simulink model "model"  (R2023b)
settings: Solver=VariableStepAuto  StartTime=0.0  StopTime=10.0  RelTol=1e-3
undefined symbols (not defined in the file): DiscIntNeverNeededParam, Newton, Raphson
libraries: simulink x46, slpidlib x9
(part 1 of 2)
settings Model: Creator=OSCAR4  LastModifiedBy=ojiken

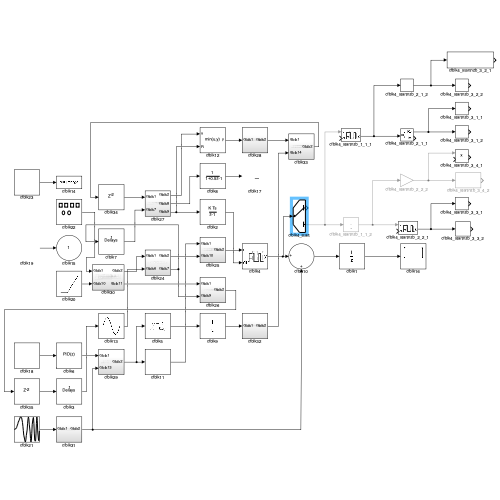
[thumbnail: Simulink's stored preview of the top-level diagram]
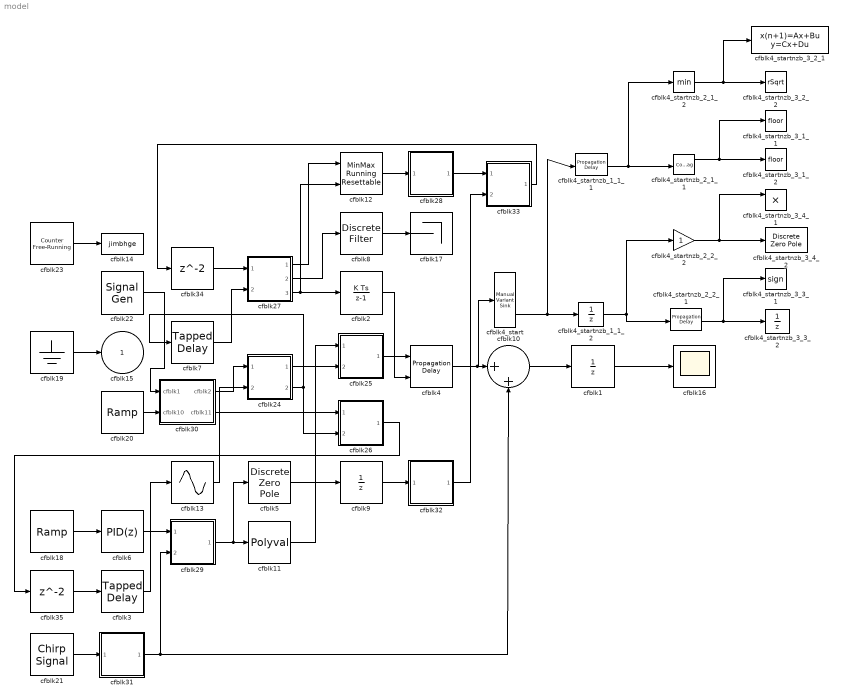
== system model ==
  cfblk1 : UnitDelay  HasFrameUpgradeWarning=on
  cfblk10 : Sum  Inputs=|++
  cfblk11 : Polyval  Coefs=[ +2.081618890e-019, -1.441693666e-014, +4.719686976e-010, -8.536869453e-006, +1.621573104e-001, -8.087801117e+001 ]
  cfblk12 : simulink/Math Operations/MinMax Running Resettable  Function=min  vinit=0.0
  cfblk13 : Sin  TimeSource=Use external signal  SampleTime=0
  cfblk14 : ToWorkspace  VariableName=jimbhge  SaveFormat=Timeseries  SampleTime=-1
  cfblk16 : Scope
  cfblk17 : Terminator
  cfblk18 : simulink/Sources/Ramp  slope=[-2549.980558]  start=[17.465354]  InitialOutput=[-530304.181969]
  cfblk19 : Ground
  cfblk2 : DiscreteIntegrator  ICPrevOutput=DiscIntNeverNeededParam  ICPrevScaledInput=DiscIntNeverNeededParam
  cfblk20 : simulink/Sources/Ramp  slope=[-906.393832]  start=[32.590534]  InitialOutput=[-89709.593460]
  cfblk21 : simulink/Sources/Chirp Signal  f1=[-269408375.768140]  T=[449577602.618100]  f2=[513643187.396250]
  cfblk22 : SignalGenerator  WaveForm=square  Amplitude=[544340339.779621]
  cfblk23 : simulink/Sources/Counter Free-Running  NumBits=[42.000000]  tsamp=-1
  cfblk24 : Subsystem
  cfblk25 : Subsystem
  cfblk26 : Subsystem
  cfblk27 : Subsystem
  cfblk28 : Subsystem
  cfblk29 : Subsystem
  cfblk3 : simulink/Discrete/Tapped Delay  vinit=0.0  samptime=-1  NumDelays=1  DelayOrder=Oldest  includeCurrent=off
  cfblk30 : Subsystem
  cfblk31 : Subsystem
  cfblk32 : Subsystem
  cfblk33 : Subsystem
  cfblk34 : Delay  SampleTime=1
  cfblk35 : Delay  SampleTime=1
  cfblk4 : PropagationDelay  SampleTime=1
  cfblk4_start : simulink/Signal Routing/Manual Variant Sink  NumChoices=2  LabelModeActiveChoice=V_1
  cfblk4_startnzb_1_1_1 : PropagationDelay
  cfblk4_startnzb_1_1_2 : UnitDelay  SampleTime=-1  HasFrameUpgradeWarning=on
  cfblk4_startnzb_2_1_1 : ComplexToRealImag
  cfblk4_startnzb_2_1_2 : MinMax
  cfblk4_startnzb_2_2_1 : PropagationDelay
  cfblk4_startnzb_2_2_2 : Gain
  cfblk4_startnzb_3_1_1 : Rounding
  cfblk4_startnzb_3_1_2 : Rounding
  cfblk4_startnzb_3_2_1 : DiscreteStateSpace  SampleTime=-1
  cfblk4_startnzb_3_2_2 : Sqrt  Operator=rSqrt
  cfblk4_startnzb_3_3_1 : Signum
  cfblk4_startnzb_3_3_2 : UnitDelay  SampleTime=-1  HasFrameUpgradeWarning=on
  cfblk4_startnzb_3_4_1 : Product
  cfblk4_startnzb_3_4_2 : DiscreteZeroPole  Poles=[0 0.5]  Gain=1  SampleTime=-1
  cfblk5 : DiscreteZeroPole  Poles=[0 0.5]  Gain=1
  cfblk6 : slpidlib/PID Controller  Controller=PID  Form=Parallel  TimeDomain=Discrete-time  UseExternalTs=off  SampleTime=1  IntegratorMethod=Forward Euler  FilterMethod=Forward Euler  ControllerParametersSource=internal  P=1  I=1  UseKiTs=off  D=0  N=100  UseFilter=on  TunerSelectOption=Transfer Function Based (PID Tuner App)  InitialConditionSource=internal  InitialConditionForIntegrator=0  InitialConditionForFilter=0  DifferentiatorICPrevScaledInput=0  ExternalReset=none  TrackingMode=off  Kt=1  LimitOutput=off  SatLimitsSource=internal  UpperSaturationLimit=inf  LowerSaturationLimit=-inf  LinearizeAsGain=off  AntiWindupMode=none  Kb=1  LimitIntegrator=off  UpperIntegratorSaturationLimit=inf  LowerIntegratorSaturationLimit=-inf  POutMin=[]  POutMax=[]  IOutMin=[]  IOutMax=[]  DOutMin=[]  DOutMax=[]  NOutMin=[]  NOutMax=[]  SumOutMin=[]  SumOutMax=[]  SaturationOutMin=[]  SaturationOutMax=[]  PParamMin=[]  PParamMax=[]  IParamMin=[]  IParamMax=[]  DParamMin=[]  DParamMax=[]  NParamMin=[]  NParamMax=[]  KbParamMin=[]  KbParamMax=[]  KtParamMin=[]  KtParamMax=[]  KbOutMin=[]  KbOutMax=[]  KtOutMin=[]  KtOutMax=[]  IntegratorOutMin=[]  IntegratorOutMax=[]  FilterOutMin=[]  FilterOutMax=[]  SumI1OutMin=[]  SumI1OutMax=[]  SumI2OutMin=[]  SumI2OutMax=[]  SumI3OutMin=[]  SumI3OutMax=[]  SumI4OutMin=[]  SumI4OutMax=[]  SumDOutMin=[]  SumDOutMax=[]  DifferentiatorOutMin=[]  DifferentiatorOutMax=[]  FilterDiffOutCoefMin=[]  FilterDiffOutCoefMax=[]  ReciprocalOutMin=[]  ReciprocalOutMax=[]  SumDenOutMin=[]  SumDenOutMax=[]  SumNumOutMin=[]  SumNumOutMax=[]  DivideOutMin=[]  DivideOutMax=[]  UdiffTsProdOutMin=[]  UdiffTsProdOutMax=[]  NTsProdOutMin=[]  NTsProdOutMax=[]  UintegralTsProdOutMin=[]  UintegralTsProdOutMax=[]  UngainTsProdOutMin=[]  UngainTsProdOutMax=[]  ClampingZeroOutDataTypeStr=Inherit: Inherit via back propagation  ClampingZeroOutMin=[]  ClampingZeroOutMax=[]  FilterDenConstantOutDataTypeStr=Inherit: Inherit via back propagation  FilterDenConstantOutMin=[]  FilterDenConstantOutMax=[]  PCopyOutDataTypeStr=Inherit: Inherit via back propagation  PCopyOutMin=[]  PCopyOutMax=[]  NCopyOutDataTypeStr=Inherit: Inherit via back propagation  NCopyOutMin=[]  NCopyOutMax=[]  IntegratorContinuousStateAttributes=''  IntegratorStateMustResolveToSignalObject=off  IntegratorRTWStateStorageClass=Auto  FilterContinuousStateAttributes=''  FilterStateMustResolveToSignalObject=off  FilterRTWStateStorageClass=Auto  ParallelPVariant=InternalParameters  IdealPVariant=Disabled  IVariant=InternalParameters  DVariant=InternalParameters  IntegratorVariant=Discrete  SatVariant=Disabled  AWVariant=Passthrough  PCopyVariant=Disabled  TRVariant=Disabled  FdbkBlocksVariant=Forward  IdealPFdbkVariant=Disabled  SatFdbkVariant=Disabled  DerivativeFilterVariant=ForwardEulerFilter  NVariant=InternalParameters  NCopyVariant=Disabled  FilterICVariant=InternalICsFilter  IntegratorICVariant=InternalICs  ExternalResetVariant=Disabled  TRSumVariant=Passthrough  SumFdbkVariant=Disabled  SumVariant=Sum_PID  TsampFilterVariant=InternalTs  TsampNgainVariant=Passthrough  TsampIntegralVariant=Disabled_SignalSpec  ExternalSaturationOutDataTypeStr=Inherit: Same as second input
      settings: LibrarySourceBlock=simulink/Discrete/Discrete PID Controller
  cfblk7 : simulink/Discrete/Tapped Delay  vinit=0.0  samptime=-1  NumDelays=1  DelayOrder=Oldest  includeCurrent=off
  cfblk8 : DiscreteFilter  SampleTime=1
  cfblk9 : UnitDelay  HasFrameUpgradeWarning=on
  cfblk15 : Outport
  wires:
  cfblk4_startnzb_2_2_2/1 -> cfblk4_startnzb_3_4_2/1, cfblk4_startnzb_3_4_1/1
  cfblk4_startnzb_2_1_2/1 -> cfblk4_startnzb_3_2_2/1, cfblk4_startnzb_3_2_1/1
  cfblk10/1 -> cfblk1/1
  cfblk33/1(cfblk2) -> cfblk34/1
  cfblk4_startnzb_1_1_2/1 -> cfblk4_startnzb_2_2_2/1, cfblk4_startnzb_2_2_1/1
  cfblk32/1(cfblk2) -> cfblk33/2(cfblk14)
  cfblk4/1 -> cfblk4_start/1, cfblk10/1
  cfblk28/1(cfblk2) -> cfblk33/1(cfblk1)
  cfblk9/1 -> cfblk32/1(cfblk1)
  cfblk2/1 -> cfblk4/2
  cfblk26/1(cfblk2) -> cfblk35/1
  cfblk8/1 -> cfblk17/1
  cfblk4_startnzb_1_1_1/1 -> cfblk4_startnzb_2_1_2/1, cfblk4_startnzb_2_1_1/1
  cfblk12/1 -> cfblk28/1(cfblk1)
  cfblk24/2(cfblk7) -> cfblk26/2(cfblk9), cfblk7/1
  cfblk30/2(cfblk11) -> cfblk26/1(cfblk1)
  cfblk27/2(cfblk8) -> cfblk8/1
  cfblk5/1 -> cfblk9/1
  cfblk27/3(cfblk9) -> cfblk2/1, cfblk12/2
  cfblk30/1(cfblk2) -> cfblk24/1(cfblk1)
  cfblk4_start/2 -> cfblk4_startnzb_1_1_2/1, cfblk4_startnzb_1_1_1/1
  cfblk7/1 -> cfblk27/2(cfblk7)
  cfblk4_startnzb_2_2_1/1 -> cfblk4_startnzb_3_3_2/1, cfblk4_startnzb_3_3_1/1
  cfblk24/1(cfblk2) -> cfblk25/2(cfblk10)
  cfblk34/1 -> cfblk27/1(cfblk1)
  cfblk20/1 -> cfblk30/2(cfblk10)
  cfblk13/1 -> cfblk24/2(cfblk6)
  cfblk18/1 -> cfblk6/1
  cfblk6/1 -> cfblk29/1(cfblk1)
  cfblk31/1(cfblk2) -> cfblk29/2(cfblk13), cfblk10/2
  cfblk23/1 -> cfblk14/1
  cfblk22/1 -> cfblk30/1(cfblk1)
  cfblk3/1 -> cfblk13/1
  cfblk27/1(cfblk2) -> cfblk12/1
  cfblk4_startnzb_2_1_1/1 -> cfblk4_startnzb_3_1_2/1, cfblk4_startnzb_3_1_1/1
  cfblk21/1 -> cfblk31/1(cfblk1)
  cfblk25/1(cfblk2) -> cfblk4/1
  cfblk35/1 -> cfblk3/1
  cfblk29/1(cfblk2) -> cfblk5/1, cfblk11/1
  cfblk19/1 -> cfblk15/1
  cfblk1/1 -> cfblk16/1
  cfblk11/1 -> cfblk25/1(cfblk1)

== system model/cfblk24 ==
  cfblk1 : Inport
  cfblk6 : Inport  Port=2
  cfblk3 : DiscreteFir  SampleTime=1
  cfblk4 : Constant  Value=[619260692.211267]  SampleTime=1
  cfblk5 : Constant  Value=[619560780.626358]  SampleTime=1
  cfblk2 : Outport
  cfblk7 : Outport  Port=2
  wires:
  cfblk6/1 -> cfblk3/1
  cfblk3/1 -> cfblk7/1
  cfblk4/1 -> cfblk2/1

== system model/cfblk25 ==
  cfblk1 : Inport
  cfblk10 : Inport  Port=2
  cfblk{11..14} (4 alike) : Delay  SampleTime=1
  cfblk3 : simulink/Discrete/Transfer Fcn Real Zero  ZeroZ=0.75  ICPrevInput=0.0  DoSatur=off
  cfblk4 : UnaryMinus
  cfblk5 : Subsystem
  cfblk6 : Subsystem
  cfblk7 : Subsystem
  cfblk8 : Subsystem
  cfblk9 : Subsystem
  cfblk2 : Outport
  wires:
  cfblk10/1 -> cfblk5/1(cfblk1)
  cfblk6/1(cfblk2) -> cfblk2/1, cfblk13/1
  cfblk8/2(cfblk11) -> cfblk3/1
  cfblk1/1 -> cfblk7/1(cfblk1), cfblk5/5(cfblk15)
  cfblk7/1(cfblk2) -> cfblk5/4(cfblk14), cfblk8/3(cfblk10)
  cfblk5/1(cfblk2) -> cfblk4/1
  cfblk4/1 -> cfblk8/1(cfblk1)
  cfblk9/1(cfblk2) -> cfblk6/1(cfblk1)
  cfblk3/1 -> cfblk9/1(cfblk1), cfblk12/1
  cfblk8/1(cfblk2) -> cfblk11/1
  cfblk11/1 -> cfblk5/3(cfblk13)
  cfblk12/1 -> cfblk8/2(cfblk9)
  cfblk13/1 -> cfblk5/2(cfblk12)
  cfblk5/2(cfblk16) -> cfblk14/1
  cfblk14/1 -> cfblk7/2(cfblk13)

== system model/cfblk26 ==
  cfblk1 : Inport
  cfblk9 : Inport  Port=2
  cfblk10 : Delay  SampleTime=1
  cfblk3 : DiscreteFilter  SampleTime=1
  cfblk4 : DiscreteIntegrator  ICPrevOutput=DiscIntNeverNeededParam  ICPrevScaledInput=DiscIntNeverNeededParam
  cfblk5 : simulink/Discrete/Transfer Fcn Real Zero  ZeroZ=0.75  ICPrevInput=0.0  DoSatur=off
  cfblk6 : Sum  Inputs=+-
  cfblk7 : Constant  Value=[-48546722.892624]  SampleTime=1
  cfblk8 : Subsystem
  cfblk2 : Outport
  wires:
  cfblk7/1 -> cfblk3/1
  cfblk3/1 -> cfblk8/1(cfblk1)
  cfblk9/1 -> cfblk4/1, cfblk8/4(cfblk13)
  cfblk4/1 -> cfblk6/1
  cfblk1/1 -> cfblk8/2(cfblk11)
  cfblk5/1 -> cfblk6/2
  cfblk8/1(cfblk2) -> cfblk5/1
  cfblk8/2(cfblk14) -> cfblk2/1
  cfblk6/1 -> cfblk10/1
  cfblk10/1 -> cfblk8/3(cfblk12)

== system model/cfblk27 ==
  cfblk1 : Inport
  cfblk7 : Inport  Port=2
  cfblk10 : Delay  SampleTime=1
  cfblk11 : Delay  SampleTime=1
  cfblk3 : Product  Inputs=*
  cfblk4 : Constant  Value=[-592211525.681612]  SampleTime=1
  cfblk5 : Subsystem
  cfblk6 : Subsystem
  cfblk2 : Outport
  cfblk8 : Outport  Port=2
  cfblk9 : Outport  Port=3
  wires:
  cfblk6/1(cfblk2) -> cfblk9/1
  cfblk7/1 -> cfblk2/1, cfblk8/1, cfblk6/3(cfblk12)
  cfblk5/1(cfblk2) -> cfblk3/1
  cfblk4/1 -> cfblk5/1(cfblk1), cfblk5/4(cfblk15), cfblk6/4(cfblk13)
  cfblk3/1 -> cfblk10/1, cfblk11/1
  cfblk1/1 -> cfblk6/2(cfblk11), cfblk5/6(cfblk17)
  cfblk6/2(cfblk15) -> cfblk5/2(cfblk13)
  cfblk6/3(cfblk16) -> cfblk5/3(cfblk14), cfblk5/5(cfblk16)
  cfblk10/1 -> cfblk6/1(cfblk1)
  cfblk11/1 -> cfblk6/5(cfblk14)

== system model/cfblk28 ==
  cfblk1 : Inport
  cfblk10 : Subsystem
  cfblk11 : Subsystem
  cfblk{12..15} (4 alike) : Delay  SampleTime=1
  cfblk3 : Delay  DelayLengthSource=Input port  SampleTime=1
      settings: InputPortMap=u0,p1
  cfblk4 : UnitDelay  HasFrameUpgradeWarning=on
  cfblk5 : Rounding
  cfblk6 : MinMax  Inputs=3
  cfblk7 : DotProduct  OutDataTypeStr=Inherit: Inherit via internal rule
  cfblk8 : Product  Inputs=**
  cfblk9 : Constant  Value=[-543142463.220039]  SampleTime=1
  cfblk2 : Outport
  wires:
  cfblk1/1 -> cfblk6/1
  cfblk9/1 -> cfblk10/1(cfblk1), cfblk11/1(cfblk1), cfblk11/3(cfblk13)
  cfblk3/1 -> cfblk10/2(cfblk14), cfblk2/1
  cfblk5/1 -> cfblk10/4(cfblk16), cfblk14/1
  cfblk6/1 -> cfblk8/2, cfblk3/1
  cfblk11/1(cfblk2) -> cfblk5/1, cfblk3/2, cfblk13/1
  cfblk8/1 -> cfblk4/1, cfblk11/2(cfblk12)
  cfblk10/1(cfblk2) -> cfblk7/1
  cfblk10/2(cfblk17) -> cfblk7/2
  cfblk4/1 -> cfblk12/1
  cfblk12/1 -> cfblk6/2
  cfblk13/1 -> cfblk6/3
  cfblk14/1 -> cfblk8/1
  cfblk7/1 -> cfblk15/1
  cfblk15/1 -> cfblk10/3(cfblk15)

== system model/cfblk29 ==
  cfblk1 : Inport
  cfblk13 : Inport  Port=2
  cfblk10 : Constant  Value=[-634116043.235819]  SampleTime=1
  cfblk11 : Subsystem
  cfblk12 : Subsystem
  cfblk14 : Delay  SampleTime=1
  cfblk3 : DiscreteFir  SampleTime=1
  cfblk4 : DiscreteStateSpace
  cfblk5 : simulink/Discrete/Transfer Fcn Lead or Lag  PoleZ=0.95  ZeroZ=0.75  ICPrevOutput=0.0  ICPrevInput=0.0  DoSatur=off
  cfblk6 : simulink/Math Operations/Slider Gain  gain=1  low=0  high=2
  cfblk7 : ComplexToRealImag
  cfblk8 : Squeeze
  cfblk9 : ComplexToMagnitudeAngle
  cfblk2 : Outport
  wires:
  cfblk4/1 -> cfblk2/1
  cfblk11/1(cfblk2) -> cfblk8/1
  cfblk7/1 -> cfblk12/1(cfblk1)
  cfblk10/1 -> cfblk5/1
  cfblk7/2 -> cfblk11/1(cfblk1)
  cfblk8/1 -> cfblk9/1
  cfblk3/1 -> cfblk7/1
  cfblk5/1 -> cfblk6/1
  cfblk9/1 -> cfblk4/1
  cfblk6/1 -> cfblk3/1
  cfblk12/1(cfblk2) -> cfblk11/3(cfblk8)
  cfblk9/2 -> cfblk14/1
  cfblk14/1 -> cfblk11/2(cfblk7)

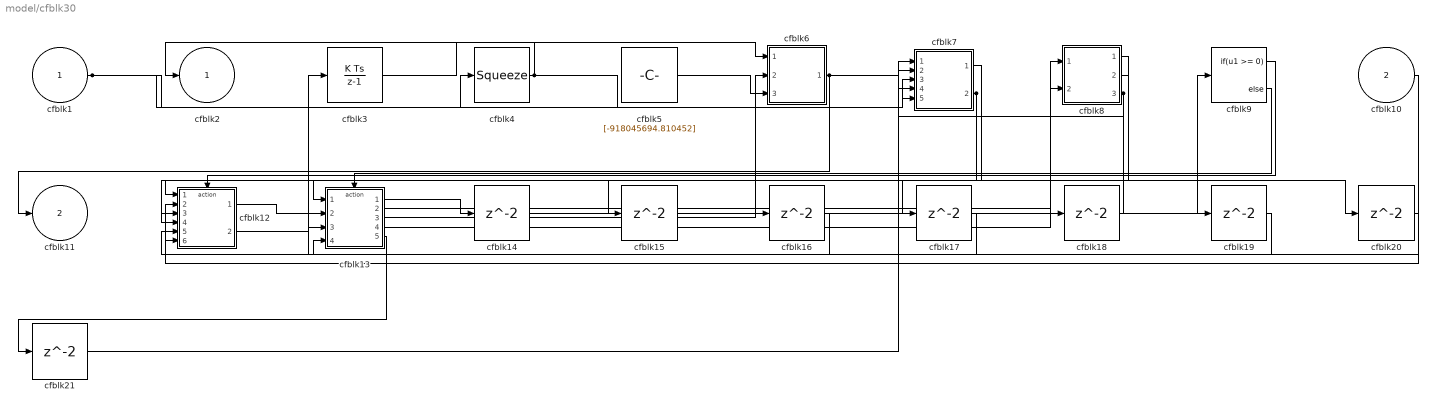
== system model/cfblk30 ==
  cfblk1 : Inport
  cfblk10 : Inport  Port=2
  cfblk12 : Subsystem  TreatAsAtomicUnit=on
  cfblk13 : Subsystem  TreatAsAtomicUnit=on
  cfblk{14..21} (8 alike) : Delay  SampleTime=1
  cfblk3 : DiscreteIntegrator  ICPrevOutput=DiscIntNeverNeededParam  ICPrevScaledInput=DiscIntNeverNeededParam
  cfblk4 : Squeeze
  cfblk5 : Constant  Value=[-918045694.810452]  SampleTime=1
  cfblk6 : Subsystem
  cfblk7 : Subsystem
  cfblk8 : Subsystem
  cfblk9 : If  IfExpression=u1 >= 0  SampleTime=1
  cfblk2 : Outport
  cfblk11 : Outport  Port=2
  wires:
  cfblk7/1(cfblk2) -> cfblk12/1(cfblk1)
  cfblk6/1(cfblk2) -> cfblk11/1, cfblk19/1, cfblk20/1
  cfblk4/1 -> cfblk2/1, cfblk7/3(cfblk13)
  cfblk7/2(cfblk16) -> cfblk13/1(cfblk1), cfblk12/3(cfblk11), cfblk12/4(cfblk12)
  cfblk1/1 -> cfblk4/1, cfblk7/5(cfblk15)
  cfblk3/1 -> cfblk6/1(cfblk1)
  cfblk13/2(cfblk14) -> cfblk8/1(cfblk1)
  cfblk13/3(cfblk15) -> cfblk6/2(cfblk10)
  cfblk5/1 -> cfblk6/3(cfblk11)
  cfblk12/1(cfblk2) -> cfblk13/2(cfblk11)
  cfblk12/2(cfblk15) -> cfblk3/1
  cfblk13/4(cfblk16) -> cfblk8/2(cfblk13)
  cfblk8/3(cfblk15) -> cfblk17/1, cfblk18/1
  cfblk10/1 -> cfblk12/2(cfblk10)
  cfblk9/1 -> cfblk12/Action
  cfblk9/2 -> cfblk13/Action
  cfblk13/1(cfblk2) -> cfblk14/1
  cfblk14/1 -> cfblk7/1(cfblk1)
  cfblk8/1(cfblk2) -> cfblk15/1
  cfblk15/1 -> cfblk9/1
  cfblk8/2(cfblk14) -> cfblk16/1
  cfblk16/1 -> cfblk13/3(cfblk12)
  cfblk17/1 -> cfblk13/4(cfblk13)
  cfblk18/1 -> cfblk7/4(cfblk14)
  cfblk19/1 -> cfblk12/5(cfblk13)
  cfblk20/1 -> cfblk12/6(cfblk14)
  cfblk13/5(cfblk17) -> cfblk21/1
  cfblk21/1 -> cfblk7/2(cfblk12)

== system model/cfblk31 ==
  cfblk1 : Inport
  cfblk3 : DiscreteFilter  SampleTime=1
  cfblk4 : simulink/Discrete/Tapped Delay  vinit=0.0  samptime=-1  NumDelays=1  DelayOrder=Oldest  includeCurrent=off
  cfblk5 : simulink/Discrete/Difference  ICPrevInput=0.0  OutMin=[]  OutMax=[]  OutDataTypeStr=Inherit: Inherit via back propagation  OutDataType=fixdt(1, 16)  OutScaling=2^-10  DoSatur=off
  cfblk6 : DiscreteFir  SampleTime=1
  cfblk7 : Math  Operator=pow
  cfblk8 : Product  Inputs=*
  cfblk2 : Outport
  wires:
  cfblk4/1 -> cfblk7/1
  cfblk1/1 -> cfblk6/1
  cfblk5/1 -> cfblk4/1
  cfblk6/1 -> cfblk5/1, cfblk3/1
  cfblk7/1 -> cfblk8/1
  cfblk8/1 -> cfblk2/1
  cfblk3/1 -> cfblk7/2

== system model/cfblk32 ==
  cfblk1 : Inport
  cfblk10 : Subsystem
  cfblk11 : Subsystem
  cfblk12 : Delay  SampleTime=1
  cfblk13 : Delay  SampleTime=1
  cfblk14 : Delay  SampleTime=1
  cfblk3 : simulink/Discrete/Transfer Fcn Lead or Lag  PoleZ=0.95  ZeroZ=0.75  ICPrevOutput=0.0  ICPrevInput=0.0  DoSatur=off
  cfblk4 : DotProduct  OutDataTypeStr=Inherit: Inherit via internal rule
  cfblk5 : Gain  Gain=[-290399110.976152]
  cfblk6 : Sin  TimeSource=Use external signal  SampleTime=0
  cfblk7 : Constant  Value=[164625169.803673]  SampleTime=1
  cfblk8 : Constant  Value=[629483974.627171]  SampleTime=1
  cfblk9 : Subsystem
  cfblk2 : Outport
  wires:
  cfblk9/1(cfblk2) -> cfblk6/1
  cfblk10/1(cfblk2) -> cfblk11/1(cfblk1)
  cfblk3/1 -> cfblk13/1, cfblk14/1
  cfblk10/2(cfblk17) -> cfblk11/3(cfblk7)
  cfblk11/1(cfblk2) -> cfblk3/1
  cfblk7/1 -> cfblk4/1, cfblk9/4(cfblk11), cfblk10/3(cfblk12), cfblk10/6(cfblk15)
  cfblk4/1 -> cfblk5/1, cfblk10/4(cfblk13)
  cfblk9/2(cfblk12) -> cfblk10/1(cfblk1)
  cfblk5/1 -> cfblk2/1
  cfblk8/1 -> cfblk9/2(cfblk9)
  cfblk1/1 -> cfblk9/3(cfblk10), cfblk10/7(cfblk16)
  cfblk9/3(cfblk13) -> cfblk4/2
  cfblk9/4(cfblk14) -> cfblk10/2(cfblk11)
  cfblk6/1 -> cfblk12/1
  cfblk12/1 -> cfblk9/1(cfblk1)
  cfblk13/1 -> cfblk11/2(cfblk6)
  cfblk14/1 -> cfblk10/5(cfblk14)

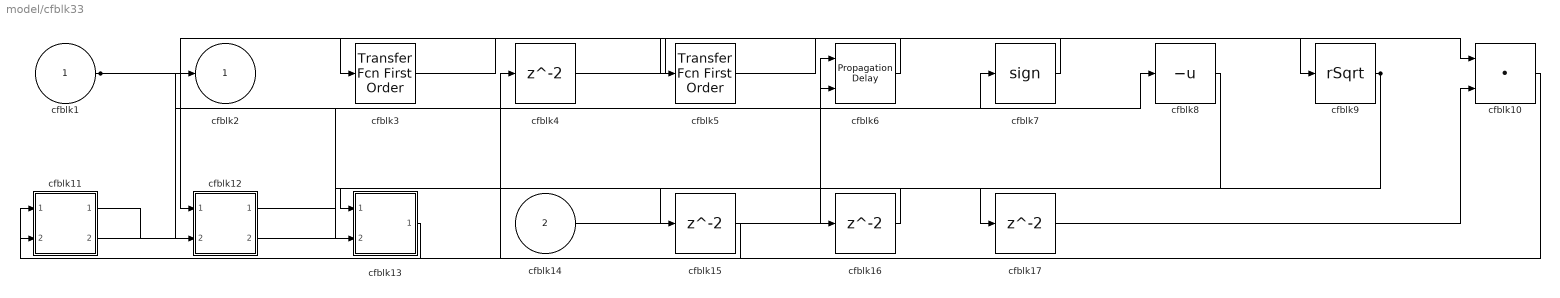
== system model/cfblk33 ==
  cfblk1 : Inport
  cfblk14 : Inport  Port=2
  cfblk10 : DotProduct  OutDataTypeStr=Inherit: Inherit via internal rule
  cfblk11 : Subsystem
  cfblk12 : Subsystem
  cfblk13 : Subsystem
  cfblk{4,15..17} (4 alike) : Delay  SampleTime=1
  cfblk3 : simulink/Discrete/Transfer Fcn First Order  PoleZ=0.95  ICPrevOutput=0.0  DoSatur=off
  cfblk5 : simulink/Discrete/Transfer Fcn First Order  PoleZ=0.95  ICPrevOutput=0.0  DoSatur=off
  cfblk6 : PropagationDelay  SampleTime=1
  cfblk7 : Signum
  cfblk8 : UnaryMinus
  cfblk9 : Sqrt  Operator=rSqrt  AlgorithmType=Newton-Raphson
  cfblk2 : Outport
  wires:
  cfblk14/1 -> cfblk6/1
  cfblk7/1 -> cfblk12/1(cfblk1)
  cfblk10/1 -> cfblk4/1
  cfblk6/1 -> cfblk3/1
  cfblk5/1 -> cfblk10/1
  cfblk4/1 -> cfblk9/1
  cfblk11/1(cfblk2) -> cfblk12/2(cfblk13)
  cfblk1/1 -> cfblk2/1, cfblk6/2
  cfblk11/2(cfblk7) -> cfblk7/1
  cfblk13/1(cfblk2) -> cfblk11/1(cfblk1)
  cfblk3/1 -> cfblk5/1
  cfblk12/2(cfblk14) -> cfblk8/1
  cfblk9/1 -> cfblk13/2(cfblk7), cfblk17/1
  cfblk12/1(cfblk2) -> cfblk15/1
  cfblk15/1 -> cfblk11/2(cfblk6)
  cfblk8/1 -> cfblk16/1
  cfblk16/1 -> cfblk13/1(cfblk1)
  cfblk17/1 -> cfblk10/2

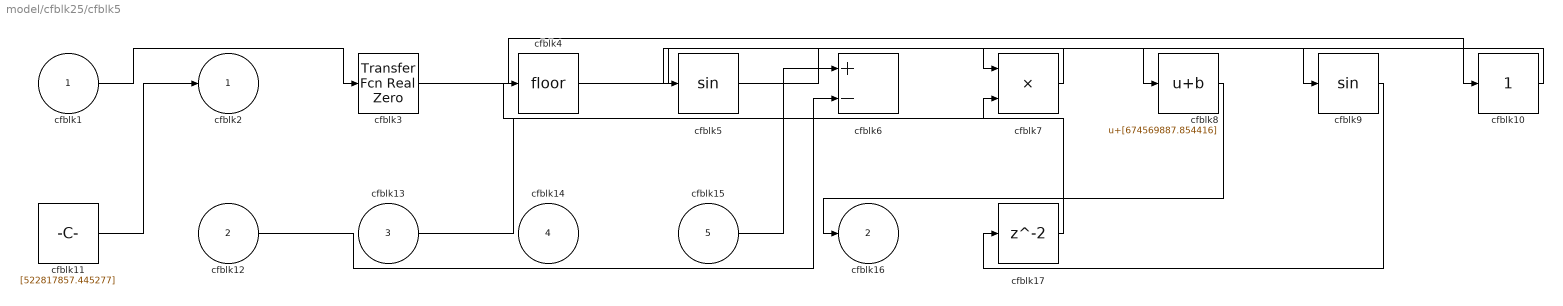
== system model/cfblk25/cfblk5 ==
  cfblk1 : Inport
  cfblk12 : Inport  Port=2
  cfblk13 : Inport  Port=3
  cfblk14 : Inport  Port=4
  cfblk15 : Inport  Port=5
  cfblk10 : simulink/Math Operations/Slider Gain  gain=1  low=0  high=2
  cfblk11 : Constant  Value=[522817857.445277]  SampleTime=1
  cfblk17 : Delay  SampleTime=1
  cfblk3 : simulink/Discrete/Transfer Fcn Real Zero  ZeroZ=0.75  ICPrevInput=0.0  DoSatur=off
  cfblk4 : Rounding
  cfblk5 : Trigonometry
  cfblk6 : Sum  Inputs=+-
  cfblk7 : Product
  cfblk8 : Bias  Bias=[674569887.854416]  SaturateOnIntegerOverflow=off
  cfblk9 : Trigonometry
  cfblk2 : Outport
  cfblk16 : Outport  Port=2
  wires:
  cfblk4/1 -> cfblk9/1
  cfblk11/1 -> cfblk2/1
  cfblk1/1 -> cfblk3/1
  cfblk15/1 -> cfblk6/1
  cfblk3/1 -> cfblk10/1
  cfblk7/1 -> cfblk5/1
  cfblk8/1 -> cfblk16/1
  cfblk12/1 -> cfblk6/2
  cfblk10/1 -> cfblk7/1
  cfblk13/1 -> cfblk7/2
  cfblk5/1 -> cfblk8/1
  cfblk9/1 -> cfblk17/1
  cfblk17/1 -> cfblk4/1

== system model/cfblk25/cfblk6 ==
  cfblk1 : Inport
  cfblk3 : DiscreteFir  SampleTime=1
  cfblk4 : simulink/Discrete/Difference  ICPrevInput=0.0  OutMin=[]  OutMax=[]  OutDataTypeStr=Inherit: Inherit via back propagation  OutDataType=fixdt(1, 16)  OutScaling=2^-10  DoSatur=off
  cfblk5 : Sum  Inputs=+-
  cfblk6 : Signum
  cfblk7 : Product
  cfblk8 : Rounding
  cfblk9 : Delay  SampleTime=1
  cfblk2 : Outport
  wires:
  cfblk3/1 -> cfblk8/1, cfblk7/2
  cfblk5/1 -> cfblk6/1
  cfblk1/1 -> cfblk5/2
  cfblk6/1 -> cfblk4/1, cfblk2/1
  cfblk4/1 -> cfblk3/1
  cfblk8/1 -> cfblk7/1
  cfblk7/1 -> cfblk9/1
  cfblk9/1 -> cfblk5/1

== system model/cfblk25/cfblk7 ==
  cfblk1 : Inport
  cfblk13 : Inport  Port=2
  cfblk10 : Abs  SaturateOnIntegerOverflow=off
  cfblk11 : Product
  cfblk12 : Constant  Value=[399015118.877011]  SampleTime=1
  cfblk14 : Delay  SampleTime=1
  cfblk15 : Delay  SampleTime=1
  cfblk3 : slpidlib/PID Controller  Controller=PID  Form=Parallel  TimeDomain=Discrete-time  UseExternalTs=off  SampleTime=1  IntegratorMethod=Forward Euler  FilterMethod=Forward Euler  ControllerParametersSource=internal  P=1  I=1  UseKiTs=off  D=0  N=100  UseFilter=on  TunerSelectOption=Transfer Function Based (PID Tuner App)  InitialConditionSource=internal  InitialConditionForIntegrator=0  InitialConditionForFilter=0  DifferentiatorICPrevScaledInput=0  ExternalReset=none  TrackingMode=off  Kt=1  LimitOutput=off  SatLimitsSource=internal  UpperSaturationLimit=inf  LowerSaturationLimit=-inf  LinearizeAsGain=off  AntiWindupMode=none  Kb=1  LimitIntegrator=off  UpperIntegratorSaturationLimit=inf  LowerIntegratorSaturationLimit=-inf  POutMin=[]  POutMax=[]  IOutMin=[]  IOutMax=[]  DOutMin=[]  DOutMax=[]  NOutMin=[]  NOutMax=[]  SumOutMin=[]  SumOutMax=[]  SaturationOutMin=[]  SaturationOutMax=[]  PParamMin=[]  PParamMax=[]  IParamMin=[]  IParamMax=[]  DParamMin=[]  DParamMax=[]  NParamMin=[]  NParamMax=[]  KbParamMin=[]  KbParamMax=[]  KtParamMin=[]  KtParamMax=[]  KbOutMin=[]  KbOutMax=[]  KtOutMin=[]  KtOutMax=[]  IntegratorOutMin=[]  IntegratorOutMax=[]  FilterOutMin=[]  FilterOutMax=[]  SumI1OutMin=[]  SumI1OutMax=[]  SumI2OutMin=[]  SumI2OutMax=[]  SumI3OutMin=[]  SumI3OutMax=[]  SumI4OutMin=[]  SumI4OutMax=[]  SumDOutMin=[]  SumDOutMax=[]  DifferentiatorOutMin=[]  DifferentiatorOutMax=[]  FilterDiffOutCoefMin=[]  FilterDiffOutCoefMax=[]  ReciprocalOutMin=[]  ReciprocalOutMax=[]  SumDenOutMin=[]  SumDenOutMax=[]  SumNumOutMin=[]  SumNumOutMax=[]  DivideOutMin=[]  DivideOutMax=[]  UdiffTsProdOutMin=[]  UdiffTsProdOutMax=[]  NTsProdOutMin=[]  NTsProdOutMax=[]  UintegralTsProdOutMin=[]  UintegralTsProdOutMax=[]  UngainTsProdOutMin=[]  UngainTsProdOutMax=[]  ClampingZeroOutDataTypeStr=Inherit: Inherit via back propagation  ClampingZeroOutMin=[]  ClampingZeroOutMax=[]  FilterDenConstantOutDataTypeStr=Inherit: Inherit via back propagation  FilterDenConstantOutMin=[]  FilterDenConstantOutMax=[]  PCopyOutDataTypeStr=Inherit: Inherit via back propagation  PCopyOutMin=[]  PCopyOutMax=[]  NCopyOutDataTypeStr=Inherit: Inherit via back propagation  NCopyOutMin=[]  NCopyOutMax=[]  IntegratorContinuousStateAttributes=''  IntegratorStateMustResolveToSignalObject=off  IntegratorRTWStateStorageClass=Auto  FilterContinuousStateAttributes=''  FilterStateMustResolveToSignalObject=off  FilterRTWStateStorageClass=Auto  ParallelPVariant=InternalParameters  IdealPVariant=Disabled  IVariant=InternalParameters  DVariant=InternalParameters  IntegratorVariant=Discrete  SatVariant=Disabled  AWVariant=Passthrough  PCopyVariant=Disabled  TRVariant=Disabled  FdbkBlocksVariant=Forward  IdealPFdbkVariant=Disabled  SatFdbkVariant=Disabled  DerivativeFilterVariant=ForwardEulerFilter  NVariant=InternalParameters  NCopyVariant=Disabled  FilterICVariant=InternalICsFilter  IntegratorICVariant=InternalICs  ExternalResetVariant=Disabled  TRSumVariant=Passthrough  SumFdbkVariant=Disabled  SumVariant=Sum_PID  TsampFilterVariant=InternalTs  TsampNgainVariant=Passthrough  TsampIntegralVariant=Disabled_SignalSpec  ExternalSaturationOutDataTypeStr=Inherit: Same as second input
      settings: LibrarySourceBlock=simulink/Discrete/Discrete PID Controller
  cfblk4 : simulink/Discrete/Transfer Fcn Lead or Lag  PoleZ=0.95  ZeroZ=0.75  ICPrevOutput=0.0  ICPrevInput=0.0  DoSatur=off
  cfblk5 : simulink/Discrete/Tapped Delay  vinit=0.0  samptime=-1  NumDelays=1  DelayOrder=Oldest  includeCurrent=off
  cfblk6 : Product
  cfblk7 : Product  Inputs=**
  cfblk8 : Sqrt  Operator=rSqrt  AlgorithmType=Newton-Raphson
  cfblk9 : Product  Inputs=**
  cfblk2 : Outport
  wires:
  cfblk3/1 -> cfblk10/1
  cfblk9/1 -> cfblk11/1
  cfblk10/1 -> cfblk7/1
  cfblk12/1 -> cfblk3/1
  cfblk1/1 -> cfblk6/1
  cfblk11/1 -> cfblk4/1
  cfblk4/1 -> cfblk7/2, cfblk15/1
  cfblk6/1 -> cfblk9/1
  cfblk5/1 -> cfblk8/1
  cfblk7/1 -> cfblk2/1, cfblk14/1
  cfblk8/1 -> cfblk9/2
  cfblk13/1 -> cfblk5/1
  cfblk14/1 -> cfblk6/2
  cfblk15/1 -> cfblk11/2

== system model/cfblk25/cfblk8 ==
  cfblk1 : Inport
  cfblk9 : Inport  Port=2
  cfblk10 : Inport  Port=3
  cfblk3 : simulink/Discrete/Tapped Delay  vinit=0.0  samptime=-1  NumDelays=1  DelayOrder=Oldest  includeCurrent=off
  cfblk4 : simulink/Discrete/Transfer Fcn Lead or Lag  PoleZ=0.95  ZeroZ=0.75  ICPrevOutput=0.0  ICPrevInput=0.0  DoSatur=off
  cfblk5 : PermuteDimensions
  cfblk6 : Signum
  cfblk7 : Constant  Value=[497245692.108561]  SampleTime=1
  cfblk8 : Constant  Value=[-352505690.659076]  SampleTime=1
  cfblk2 : Outport
  cfblk11 : Outport  Port=2
  wires:
  cfblk3/1 -> cfblk2/1
  cfblk9/1 -> cfblk4/1
  cfblk1/1 -> cfblk5/1
  cfblk4/1 -> cfblk6/1
  cfblk10/1 -> cfblk11/1
  cfblk7/1 -> cfblk3/1

== system model/cfblk25/cfblk9 ==
  cfblk1 : Inport
  cfblk10 : UnaryMinus
  cfblk11 : simulink/Math Operations/MinMax Running Resettable  Function=min  vinit=0.0
  cfblk12 : Constant  Value=[-589662599.305054]  SampleTime=1
  cfblk13 : Constant  Value=[-897290192.026509]  SampleTime=1
  cfblk14 : Constant  Value=[-404888619.665667]  SampleTime=1
  cfblk15 : Delay  SampleTime=1
  cfblk3 : UnitDelay  HasFrameUpgradeWarning=on
  cfblk4 : slpidlib/PID Controller (2DOF)  Controller=PID  Form=Parallel  TimeDomain=Discrete-time  UseExternalTs=off  SampleTime=1  IntegratorMethod=Forward Euler  FilterMethod=Forward Euler  ControllerParametersSource=internal  P=1  I=1  UseKiTs=off  D=0  N=100  UseFilter=on  b=1  c=1  TunerSelectOption=Transfer Function Based (PID Tuner App)  InitialConditionSource=internal  InitialConditionForIntegrator=0  InitialConditionForFilter=0  DifferentiatorICPrevScaledInput=0  ExternalReset=none  TrackingMode=off  Kt=1  LimitOutput=off  SatLimitsSource=internal  UpperSaturationLimit=inf  LowerSaturationLimit=-inf  LinearizeAsGain=off  AntiWindupMode=none  Kb=1  LimitIntegrator=off  UpperIntegratorSaturationLimit=inf  LowerIntegratorSaturationLimit=-inf  POutMin=[]  POutMax=[]  IOutMin=[]  IOutMax=[]  DOutMin=[]  DOutMax=[]  NOutMin=[]  NOutMax=[]  bOutMin=[]  bOutMax=[]  cOutMin=[]  cOutMax=[]  SumOutMin=[]  SumOutMax=[]  SaturationOutMin=[]  SaturationOutMax=[]  PParamMin=[]  PParamMax=[]  IParamMin=[]  IParamMax=[]  DParamMin=[]  DParamMax=[]  NParamMin=[]  NParamMax=[]  bParamMin=[]  bParamMax=[]  cParamMin=[]  cParamMax=[]  KbParamMin=[]  KbParamMax=[]  KtParamMin=[]  KtParamMax=[]  KbOutMin=[]  KbOutMax=[]  KtOutMin=[]  KtOutMax=[]  IntegratorOutMin=[]  IntegratorOutMax=[]  FilterOutMin=[]  FilterOutMax=[]  SumI1OutMin=[]  SumI1OutMax=[]  SumI2OutMin=[]  SumI2OutMax=[]  SumI3OutMin=[]  SumI3OutMax=[]  SumI4OutMin=[]  SumI4OutMax=[]  SumDOutMin=[]  SumDOutMax=[]  Sum1OutMin=[]  Sum1OutMax=[]  Sum2OutMin=[]  Sum2OutMax=[]  Sum3OutMin=[]  Sum3OutMax=[]  DifferentiatorOutMin=[]  DifferentiatorOutMax=[]  FilterDiffOutCoefMin=[]  FilterDiffOutCoefMax=[]  ReciprocalOutMin=[]  ReciprocalOutMax=[]  SumDenOutMin=[]  SumDenOutMax=[]  SumNumOutMin=[]  SumNumOutMax=[]  DivideOutMin=[]  DivideOutMax=[]  UdiffTsProdOutMin=[]  UdiffTsProdOutMax=[]  NTsProdOutMin=[]  NTsProdOutMax=[]  UintegralTsProdOutMin=[]  UintegralTsProdOutMax=[]  UngainTsProdOutMin=[]  UngainTsProdOutMax=[]  ClampingZeroOutDataTypeStr=Inherit: Inherit via back propagation  ClampingZeroOutMin=[]  ClampingZeroOutMax=[]  FilterDenConstantOutDataTypeStr=Inherit: Inherit via back propagation  FilterDenConstantOutMin=[]  FilterDenConstantOutMax=[]  PCopyOutDataTypeStr=Inherit: Inherit via back propagation  PCopyOutMin=[]  PCopyOutMax=[]  NCopyOutDataTypeStr=Inherit: Inherit via back propagation  NCopyOutMin=[]  NCopyOutMax=[]  IntegratorContinuousStateAttributes=''  IntegratorStateMustResolveToSignalObject=off  IntegratorRTWStateStorageClass=Auto  FilterContinuousStateAttributes=''  FilterStateMustResolveToSignalObject=off  FilterRTWStateStorageClass=Auto  ParallelPVariant=InternalParameters  IdealPVariant=Disabled  IVariant=InternalParameters  DVariant=InternalParameters  bVariant=InternalParameters  cVariant=InternalParameters  IntegratorVariant=Discrete  SatVariant=Disabled  AWVariant=Passthrough  PCopyVariant=Disabled  TRVariant=Disabled  FdbkBlocksVariant=Forward  IdealPFdbkVariant=Disabled  SatFdbkVariant=Disabled  DerivativeFilterVariant=ForwardEulerFilter  NVariant=InternalParameters  NCopyVariant=Disabled  FilterICVariant=InternalICsFilter  IntegratorICVariant=InternalICs  ExternalResetVariant=Disabled  TRSumVariant=Passthrough  SumFdbkVariant=Disabled  SumVariant=Sum_PID  TsampFilterVariant=InternalTs  TsampNgainVariant=Passthrough  TsampIntegralVariant=Disabled_SignalSpec  ExternalSaturationOutDataTypeStr=Inherit: Same as second input
      settings: LibrarySourceBlock=simulink/Discrete/Discrete PID Controller (2DOF)
  cfblk5 : slpidlib/PID Controller  Controller=PID  Form=Parallel  TimeDomain=Discrete-time  UseExternalTs=off  SampleTime=1  IntegratorMethod=Forward Euler  FilterMethod=Forward Euler  ControllerParametersSource=internal  P=1  I=1  UseKiTs=off  D=0  N=100  UseFilter=on  TunerSelectOption=Transfer Function Based (PID Tuner App)  InitialConditionSource=internal  InitialConditionForIntegrator=0  InitialConditionForFilter=0  DifferentiatorICPrevScaledInput=0  ExternalReset=none  TrackingMode=off  Kt=1  LimitOutput=off  SatLimitsSource=internal  UpperSaturationLimit=inf  LowerSaturationLimit=-inf  LinearizeAsGain=off  AntiWindupMode=none  Kb=1  LimitIntegrator=off  UpperIntegratorSaturationLimit=inf  LowerIntegratorSaturationLimit=-inf  POutMin=[]  POutMax=[]  IOutMin=[]  IOutMax=[]  DOutMin=[]  DOutMax=[]  NOutMin=[]  NOutMax=[]  SumOutMin=[]  SumOutMax=[]  SaturationOutMin=[]  SaturationOutMax=[]  PParamMin=[]  PParamMax=[]  IParamMin=[]  IParamMax=[]  DParamMin=[]  DParamMax=[]  NParamMin=[]  NParamMax=[]  KbParamMin=[]  KbParamMax=[]  KtParamMin=[]  KtParamMax=[]  KbOutMin=[]  KbOutMax=[]  KtOutMin=[]  KtOutMax=[]  IntegratorOutMin=[]  IntegratorOutMax=[]  FilterOutMin=[]  FilterOutMax=[]  SumI1OutMin=[]  SumI1OutMax=[]  SumI2OutMin=[]  SumI2OutMax=[]  SumI3OutMin=[]  SumI3OutMax=[]  SumI4OutMin=[]  SumI4OutMax=[]  SumDOutMin=[]  SumDOutMax=[]  DifferentiatorOutMin=[]  DifferentiatorOutMax=[]  FilterDiffOutCoefMin=[]  FilterDiffOutCoefMax=[]  ReciprocalOutMin=[]  ReciprocalOutMax=[]  SumDenOutMin=[]  SumDenOutMax=[]  SumNumOutMin=[]  SumNumOutMax=[]  DivideOutMin=[]  DivideOutMax=[]  UdiffTsProdOutMin=[]  UdiffTsProdOutMax=[]  NTsProdOutMin=[]  NTsProdOutMax=[]  UintegralTsProdOutMin=[]  UintegralTsProdOutMax=[]  UngainTsProdOutMin=[]  UngainTsProdOutMax=[]  ClampingZeroOutDataTypeStr=Inherit: Inherit via back propagation  ClampingZeroOutMin=[]  ClampingZeroOutMax=[]  FilterDenConstantOutDataTypeStr=Inherit: Inherit via back propagation  FilterDenConstantOutMin=[]  FilterDenConstantOutMax=[]  PCopyOutDataTypeStr=Inherit: Inherit via back propagation  PCopyOutMin=[]  PCopyOutMax=[]  NCopyOutDataTypeStr=Inherit: Inherit via back propagation  NCopyOutMin=[]  NCopyOutMax=[]  IntegratorContinuousStateAttributes=''  IntegratorStateMustResolveToSignalObject=off  IntegratorRTWStateStorageClass=Auto  FilterContinuousStateAttributes=''  FilterStateMustResolveToSignalObject=off  FilterRTWStateStorageClass=Auto  ParallelPVariant=InternalParameters  IdealPVariant=Disabled  IVariant=InternalParameters  DVariant=InternalParameters  IntegratorVariant=Discrete  SatVariant=Disabled  AWVariant=Passthrough  PCopyVariant=Disabled  TRVariant=Disabled  FdbkBlocksVariant=Forward  IdealPFdbkVariant=Disabled  SatFdbkVariant=Disabled  DerivativeFilterVariant=ForwardEulerFilter  NVariant=InternalParameters  NCopyVariant=Disabled  FilterICVariant=InternalICsFilter  IntegratorICVariant=InternalICs  ExternalResetVariant=Disabled  TRSumVariant=Passthrough  SumFdbkVariant=Disabled  SumVariant=Sum_PID  TsampFilterVariant=InternalTs  TsampNgainVariant=Passthrough  TsampIntegralVariant=Disabled_SignalSpec  ExternalSaturationOutDataTypeStr=Inherit: Same as second input
      settings: LibrarySourceBlock=simulink/Discrete/Discrete PID Controller
  cfblk6 : simulink/Discrete/Tapped Delay  vinit=0.0  samptime=-1  NumDelays=1  DelayOrder=Oldest  includeCurrent=off
  cfblk7 : DiscreteTransferFcn  SampleTime=1
  cfblk8 : Sum  Inputs=+
  cfblk9 : Sqrt  Operator=rSqrt  AlgorithmType=Newton-Raphson
  cfblk2 : Outport
  wires:
  cfblk3/1 -> cfblk10/1
  cfblk4/1 -> cfblk6/1
  cfblk1/1 -> cfblk4/1
  cfblk13/1 -> cfblk8/1
  cfblk14/1 -> cfblk4/2
  cfblk8/1 -> cfblk7/1
  cfblk12/1 -> cfblk11/1
  cfblk6/1 -> cfblk11/2
  cfblk11/1 -> cfblk2/1
  cfblk7/1 -> cfblk5/1
  cfblk5/1 -> cfblk9/1
  cfblk10/1 -> cfblk15/1
  cfblk15/1 -> cfblk3/1

== system model/cfblk26/cfblk8 ==
  cfblk1 : Inport
  cfblk11 : Inport  Port=2
  cfblk12 : Inport  Port=3
  cfblk13 : Inport  Port=4
  cfblk10 : Constant  Value=[-146083815.756705]  SampleTime=1
  cfblk3 : DiscreteFir  SampleTime=1
  cfblk4 : simulink/Discrete/Transfer Fcn First Order  PoleZ=0.95  ICPrevOutput=0.0  DoSatur=off
  cfblk5 : simulink/Discrete/Tapped Delay  vinit=0.0  samptime=-1  NumDelays=1  DelayOrder=Oldest  includeCurrent=off
  cfblk6 : simulink/Discrete/Transfer Fcn First Order  PoleZ=0.95  ICPrevOutput=0.0  DoSatur=off
  cfblk7 : Sqrt
  cfblk8 : Sqrt  Operator=rSqrt  AlgorithmType=Newton-Raphson
  cfblk9 : Trigonometry
  cfblk2 : Outport
  cfblk14 : Outport  Port=2
  wires:
  cfblk10/1 -> cfblk8/1
  cfblk13/1 -> cfblk7/1
  cfblk8/1 -> cfblk2/1
  cfblk7/1 -> cfblk14/1
  cfblk1/1 -> cfblk9/1
  cfblk12/1 -> cfblk4/1
  cfblk3/1 -> cfblk6/1
  cfblk11/1 -> cfblk5/1
  cfblk4/1 -> cfblk3/1

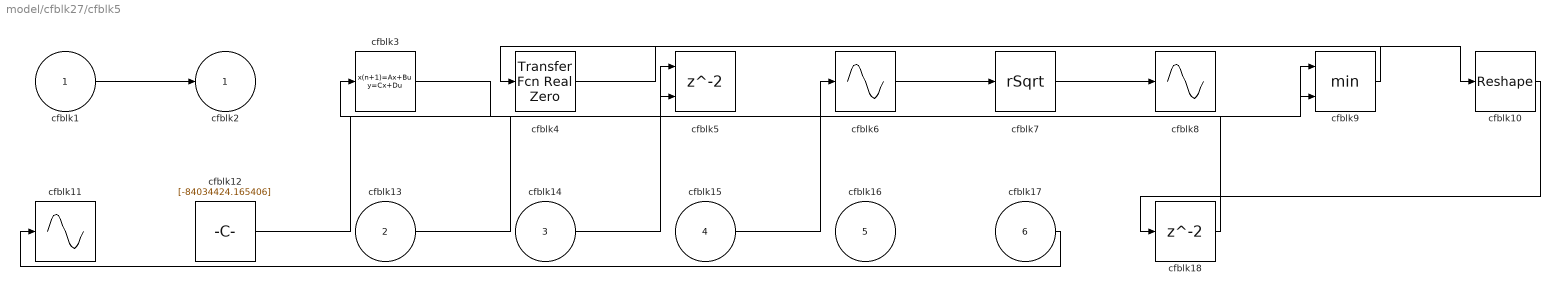
== system model/cfblk27/cfblk5 ==
  cfblk1 : Inport
  cfblk13 : Inport  Port=2
  cfblk14 : Inport  Port=3
  cfblk15 : Inport  Port=4
  cfblk16 : Inport  Port=5
  cfblk17 : Inport  Port=6
  cfblk10 : Reshape
  cfblk11 : Sin  TimeSource=Use external signal  SampleTime=0
  cfblk12 : Constant  Value=[-84034424.165406]  SampleTime=1
  cfblk18 : Delay  SampleTime=1
  cfblk3 : DiscreteStateSpace
  cfblk4 : simulink/Discrete/Transfer Fcn Real Zero  ZeroZ=0.75  ICPrevInput=0.0  DoSatur=off
  cfblk5 : Delay  ShowEnablePort=on  SampleTime=1
      settings: InputPortMap=u0,e6
  cfblk6 : Sin  TimeSource=Use external signal  SampleTime=0
  cfblk7 : Sqrt  Operator=rSqrt  AlgorithmType=Newton-Raphson
  cfblk8 : Sin  TimeSource=Use external signal  SampleTime=0
  cfblk9 : MinMax  Inputs=2
  cfblk2 : Outport
  wires:
  cfblk1/1 -> cfblk2/1
  cfblk9/1 -> cfblk4/1
  cfblk3/1 -> cfblk9/1
  cfblk15/1 -> cfblk6/1
  cfblk12/1 -> cfblk9/2
  cfblk17/1 -> cfblk11/1
  cfblk6/1 -> cfblk7/1
  cfblk13/1 -> cfblk5/1
  cfblk14/1 -> cfblk5/2
  cfblk4/1 -> cfblk10/1
  cfblk7/1 -> cfblk8/1
  cfblk10/1 -> cfblk18/1
  cfblk18/1 -> cfblk3/1

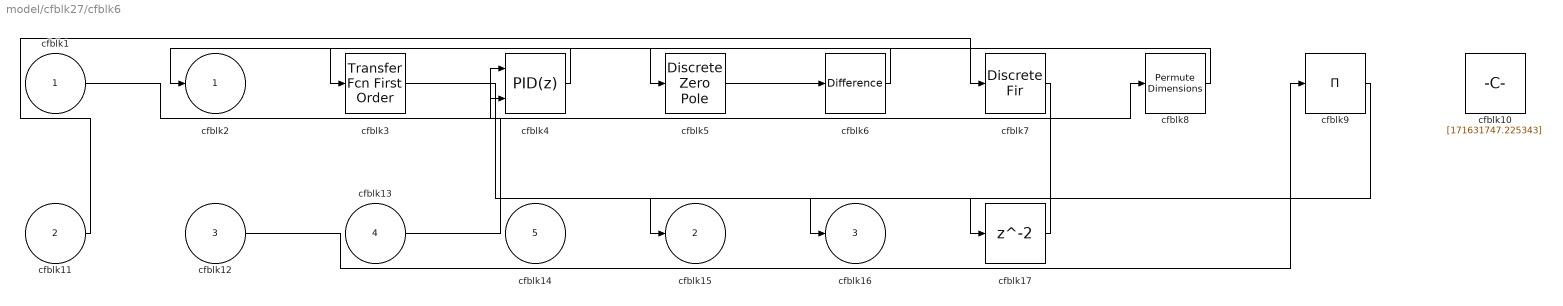
== system model/cfblk27/cfblk6 ==
  cfblk1 : Inport
  cfblk11 : Inport  Port=2
  cfblk12 : Inport  Port=3
  cfblk13 : Inport  Port=4
  cfblk14 : Inport  Port=5
  cfblk10 : Constant  Value=[171631747.225343]  SampleTime=1
  cfblk17 : Delay  SampleTime=1
  cfblk3 : simulink/Discrete/Transfer Fcn First Order  PoleZ=0.95  ICPrevOutput=0.0  DoSatur=off
  cfblk4 : slpidlib/PID Controller (2DOF)  Controller=PID  Form=Parallel  TimeDomain=Discrete-time  UseExternalTs=off  SampleTime=1  IntegratorMethod=Forward Euler  FilterMethod=Forward Euler  ControllerParametersSource=internal  P=1  I=1  UseKiTs=off  D=0  N=100  UseFilter=on  b=1  c=1  TunerSelectOption=Transfer Function Based (PID Tuner App)  InitialConditionSource=internal  InitialConditionForIntegrator=0  InitialConditionForFilter=0  DifferentiatorICPrevScaledInput=0  ExternalReset=none  TrackingMode=off  Kt=1  LimitOutput=off  SatLimitsSource=internal  UpperSaturationLimit=inf  LowerSaturationLimit=-inf  LinearizeAsGain=off  AntiWindupMode=none  Kb=1  LimitIntegrator=off  UpperIntegratorSaturationLimit=inf  LowerIntegratorSaturationLimit=-inf  POutMin=[]  POutMax=[]  IOutMin=[]  IOutMax=[]  DOutMin=[]  DOutMax=[]  NOutMin=[]  NOutMax=[]  bOutMin=[]  bOutMax=[]  cOutMin=[]  cOutMax=[]  SumOutMin=[]  SumOutMax=[]  SaturationOutMin=[]  SaturationOutMax=[]  PParamMin=[]  PParamMax=[]  IParamMin=[]  IParamMax=[]  DParamMin=[]  DParamMax=[]  NParamMin=[]  NParamMax=[]  bParamMin=[]  bParamMax=[]  cParamMin=[]  cParamMax=[]  KbParamMin=[]  KbParamMax=[]  KtParamMin=[]  KtParamMax=[]  KbOutMin=[]  KbOutMax=[]  KtOutMin=[]  KtOutMax=[]  IntegratorOutMin=[]  IntegratorOutMax=[]  FilterOutMin=[]  FilterOutMax=[]  SumI1OutMin=[]  SumI1OutMax=[]  SumI2OutMin=[]  SumI2OutMax=[]  SumI3OutMin=[]  SumI3OutMax=[]  SumI4OutMin=[]  SumI4OutMax=[]  SumDOutMin=[]  SumDOutMax=[]  Sum1OutMin=[]  Sum1OutMax=[]  Sum2OutMin=[]  Sum2OutMax=[]  Sum3OutMin=[]  Sum3OutMax=[]  DifferentiatorOutMin=[]  DifferentiatorOutMax=[]  FilterDiffOutCoefMin=[]  FilterDiffOutCoefMax=[]  ReciprocalOutMin=[]  ReciprocalOutMax=[]  SumDenOutMin=[]  SumDenOutMax=[]  SumNumOutMin=[]  SumNumOutMax=[]  DivideOutMin=[]  DivideOutMax=[]  UdiffTsProdOutMin=[]  UdiffTsProdOutMax=[]  NTsProdOutMin=[]  NTsProdOutMax=[]  UintegralTsProdOutMin=[]  UintegralTsProdOutMax=[]  UngainTsProdOutMin=[]  UngainTsProdOutMax=[]  ClampingZeroOutDataTypeStr=Inherit: Inherit via back propagation  ClampingZeroOutMin=[]  ClampingZeroOutMax=[]  FilterDenConstantOutDataTypeStr=Inherit: Inherit via back propagation  FilterDenConstantOutMin=[]  FilterDenConstantOutMax=[]  PCopyOutDataTypeStr=Inherit: Inherit via back propagation  PCopyOutMin=[]  PCopyOutMax=[]  NCopyOutDataTypeStr=Inherit: Inherit via back propagation  NCopyOutMin=[]  NCopyOutMax=[]  IntegratorContinuousStateAttributes=''  IntegratorStateMustResolveToSignalObject=off  IntegratorRTWStateStorageClass=Auto  FilterContinuousStateAttributes=''  FilterStateMustResolveToSignalObject=off  FilterRTWStateStorageClass=Auto  ParallelPVariant=InternalParameters  IdealPVariant=Disabled  IVariant=InternalParameters  DVariant=InternalParameters  bVariant=InternalParameters  cVariant=InternalParameters  IntegratorVariant=Discrete  SatVariant=Disabled  AWVariant=Passthrough  PCopyVariant=Disabled  TRVariant=Disabled  FdbkBlocksVariant=Forward  IdealPFdbkVariant=Disabled  SatFdbkVariant=Disabled  DerivativeFilterVariant=ForwardEulerFilter  NVariant=InternalParameters  NCopyVariant=Disabled  FilterICVariant=InternalICsFilter  IntegratorICVariant=InternalICs  ExternalResetVariant=Disabled  TRSumVariant=Passthrough  SumFdbkVariant=Disabled  SumVariant=Sum_PID  TsampFilterVariant=InternalTs  TsampNgainVariant=Passthrough  TsampIntegralVariant=Disabled_SignalSpec  ExternalSaturationOutDataTypeStr=Inherit: Same as second input
      settings: LibrarySourceBlock=simulink/Discrete/Discrete PID Controller (2DOF)
  cfblk5 : DiscreteZeroPole  Poles=[0 0.5]  Gain=1
  cfblk6 : simulink/Discrete/Difference  ICPrevInput=0.0  OutMin=[]  OutMax=[]  OutDataTypeStr=Inherit: Inherit via back propagation  OutDataType=fixdt(1, 16)  OutScaling=2^-10  DoSatur=off
  cfblk7 : DiscreteFir  SampleTime=1
  cfblk8 : PermuteDimensions
  cfblk9 : Product  Inputs=*
  cfblk2 : Outport
  cfblk15 : Outport  Port=2
  cfblk16 : Outport  Port=3
  wires:
  cfblk6/1 -> cfblk2/1
  cfblk13/1 -> cfblk8/1
  cfblk5/1 -> cfblk6/1
  cfblk7/1 -> cfblk15/1
  cfblk1/1 -> cfblk4/1
  cfblk4/1 -> cfblk3/1
  cfblk11/1 -> cfblk7/1
  cfblk12/1 -> cfblk9/1
  cfblk8/1 -> cfblk5/1
  cfblk9/1 -> cfblk16/1
  cfblk3/1 -> cfblk17/1
  cfblk17/1 -> cfblk4/2

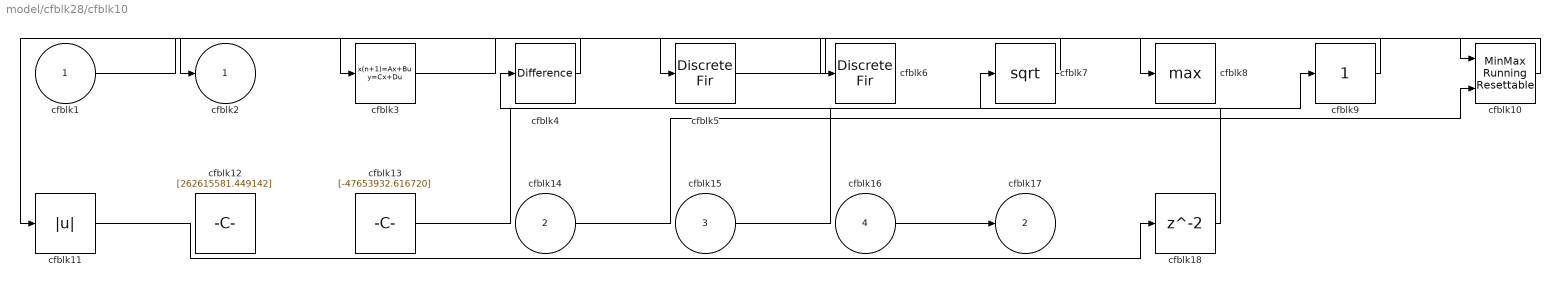
== system model/cfblk28/cfblk10 ==
  cfblk1 : Inport
  cfblk14 : Inport  Port=2
  cfblk15 : Inport  Port=3
  cfblk16 : Inport  Port=4
  cfblk10 : simulink/Math Operations/MinMax Running Resettable  Function=min  vinit=0.0
  cfblk11 : Abs  SaturateOnIntegerOverflow=off
  cfblk12 : Constant  Value=[262615581.449142]  SampleTime=1
  cfblk13 : Constant  Value=[-47653932.616720]  SampleTime=1
  cfblk18 : Delay  SampleTime=1
  cfblk3 : DiscreteStateSpace
  cfblk4 : simulink/Discrete/Difference  ICPrevInput=0.0  OutMin=[]  OutMax=[]  OutDataTypeStr=Inherit: Inherit via back propagation  OutDataType=fixdt(1, 16)  OutScaling=2^-10  DoSatur=off
  cfblk5 : DiscreteFir  SampleTime=1
  cfblk6 : DiscreteFir  SampleTime=1
  cfblk7 : Sqrt
  cfblk8 : MinMax  Function=max
  cfblk9 : simulink/Math Operations/Slider Gain  gain=1  low=0  high=2
  cfblk2 : Outport
  cfblk17 : Outport  Port=2
  wires:
  cfblk5/1 -> cfblk10/1
  cfblk13/1 -> cfblk7/1
  cfblk4/1 -> cfblk11/1
  cfblk7/1 -> cfblk5/1
  cfblk14/1 -> cfblk10/2
  cfblk15/1 -> cfblk9/1
  cfblk9/1 -> cfblk2/1
  cfblk1/1 -> cfblk6/1
  cfblk3/1 -> cfblk8/1
  cfblk10/1 -> cfblk3/1
  cfblk16/1 -> cfblk17/1
  cfblk11/1 -> cfblk18/1
  cfblk18/1 -> cfblk4/1

== system model/cfblk28/cfblk11 ==
  cfblk1 : Inport
  cfblk12 : Inport  Port=2
  cfblk13 : Inport  Port=3
  cfblk10 : Constant  Value=[146814281.342832]  SampleTime=1
  cfblk11 : Constant  Value=[557597971.327847]  SampleTime=1
  cfblk3 : simulink/Discrete/Transfer Fcn Real Zero  ZeroZ=0.75  ICPrevInput=0.0  DoSatur=off
  cfblk4 : Delay  DelayLengthSource=Input port  SampleTime=1
      settings: InputPortMap=u0,p1
  cfblk5 : Polyval  Coefs=[ +2.081618890e-019, -1.441693666e-014, +4.719686976e-010, -8.536869453e-006, +1.621573104e-001, -8.087801117e+001 ]
  cfblk6 : Signum
  cfblk7 : Reshape
  cfblk8 : Sum  Inputs=+
  cfblk9 : Constant  Value=[-502071521.517534]  SampleTime=1
  cfblk2 : Outport
  wires:
  cfblk3/1 -> cfblk7/1
  cfblk12/1 -> cfblk6/1
  cfblk8/1 -> cfblk5/1
  cfblk6/1 -> cfblk8/1
  cfblk10/1 -> cfblk3/1
  cfblk9/1 -> cfblk2/1
  cfblk5/1 -> cfblk4/1
  cfblk1/1 -> cfblk4/2

== system model/cfblk29/cfblk11 ==
  cfblk1 : Inport
  cfblk7 : Inport  Port=2
  cfblk8 : Inport  Port=3
  cfblk3 : DiscreteFilter  SampleTime=1
  cfblk4 : slpidlib/PID Controller (2DOF)  Controller=PID  Form=Parallel  TimeDomain=Discrete-time  UseExternalTs=off  SampleTime=1  IntegratorMethod=Forward Euler  FilterMethod=Forward Euler  ControllerParametersSource=internal  P=1  I=1  UseKiTs=off  D=0  N=100  UseFilter=on  b=1  c=1  TunerSelectOption=Transfer Function Based (PID Tuner App)  InitialConditionSource=internal  InitialConditionForIntegrator=0  InitialConditionForFilter=0  DifferentiatorICPrevScaledInput=0  ExternalReset=none  TrackingMode=off  Kt=1  LimitOutput=off  SatLimitsSource=internal  UpperSaturationLimit=inf  LowerSaturationLimit=-inf  LinearizeAsGain=off  AntiWindupMode=none  Kb=1  LimitIntegrator=off  UpperIntegratorSaturationLimit=inf  LowerIntegratorSaturationLimit=-inf  POutMin=[]  POutMax=[]  IOutMin=[]  IOutMax=[]  DOutMin=[]  DOutMax=[]  NOutMin=[]  NOutMax=[]  bOutMin=[]  bOutMax=[]  cOutMin=[]  cOutMax=[]  SumOutMin=[]  SumOutMax=[]  SaturationOutMin=[]  SaturationOutMax=[]  PParamMin=[]  PParamMax=[]  IParamMin=[]  IParamMax=[]  DParamMin=[]  DParamMax=[]  NParamMin=[]  NParamMax=[]  bParamMin=[]  bParamMax=[]  cParamMin=[]  cParamMax=[]  KbParamMin=[]  KbParamMax=[]  KtParamMin=[]  KtParamMax=[]  KbOutMin=[]  KbOutMax=[]  KtOutMin=[]  KtOutMax=[]  IntegratorOutMin=[]  IntegratorOutMax=[]  FilterOutMin=[]  FilterOutMax=[]  SumI1OutMin=[]  SumI1OutMax=[]  SumI2OutMin=[]  SumI2OutMax=[]  SumI3OutMin=[]  SumI3OutMax=[]  SumI4OutMin=[]  SumI4OutMax=[]  SumDOutMin=[]  SumDOutMax=[]  Sum1OutMin=[]  Sum1OutMax=[]  Sum2OutMin=[]  Sum2OutMax=[]  Sum3OutMin=[]  Sum3OutMax=[]  DifferentiatorOutMin=[]  DifferentiatorOutMax=[]  FilterDiffOutCoefMin=[]  FilterDiffOutCoefMax=[]  ReciprocalOutMin=[]  ReciprocalOutMax=[]  SumDenOutMin=[]  SumDenOutMax=[]  SumNumOutMin=[]  SumNumOutMax=[]  DivideOutMin=[]  DivideOutMax=[]  UdiffTsProdOutMin=[]  UdiffTsProdOutMax=[]  NTsProdOutMin=[]  NTsProdOutMax=[]  UintegralTsProdOutMin=[]  UintegralTsProdOutMax=[]  UngainTsProdOutMin=[]  UngainTsProdOutMax=[]  ClampingZeroOutDataTypeStr=Inherit: Inherit via back propagation  ClampingZeroOutMin=[]  ClampingZeroOutMax=[]  FilterDenConstantOutDataTypeStr=Inherit: Inherit via back propagation  FilterDenConstantOutMin=[]  FilterDenConstantOutMax=[]  PCopyOutDataTypeStr=Inherit: Inherit via back propagation  PCopyOutMin=[]  PCopyOutMax=[]  NCopyOutDataTypeStr=Inherit: Inherit via back propagation  NCopyOutMin=[]  NCopyOutMax=[]  IntegratorContinuousStateAttributes=''  IntegratorStateMustResolveToSignalObject=off  IntegratorRTWStateStorageClass=Auto  FilterContinuousStateAttributes=''  FilterStateMustResolveToSignalObject=off  FilterRTWStateStorageClass=Auto  ParallelPVariant=InternalParameters  IdealPVariant=Disabled  IVariant=InternalParameters  DVariant=InternalParameters  bVariant=InternalParameters  cVariant=InternalParameters  IntegratorVariant=Discrete  SatVariant=Disabled  AWVariant=Passthrough  PCopyVariant=Disabled  TRVariant=Disabled  FdbkBlocksVariant=Forward  IdealPFdbkVariant=Disabled  SatFdbkVariant=Disabled  DerivativeFilterVariant=ForwardEulerFilter  NVariant=InternalParameters  NCopyVariant=Disabled  FilterICVariant=InternalICsFilter  IntegratorICVariant=InternalICs  ExternalResetVariant=Disabled  TRSumVariant=Passthrough  SumFdbkVariant=Disabled  SumVariant=Sum_PID  TsampFilterVariant=InternalTs  TsampNgainVariant=Passthrough  TsampIntegralVariant=Disabled_SignalSpec  ExternalSaturationOutDataTypeStr=Inherit: Same as second input
      settings: LibrarySourceBlock=simulink/Discrete/Discrete PID Controller (2DOF)
  cfblk5 : Sum  Inputs=+-
  cfblk6 : Sqrt  Operator=rSqrt  AlgorithmType=Newton-Raphson
  cfblk9 : Delay  SampleTime=1
  cfblk2 : Outport
  wires:
  cfblk7/1 -> cfblk4/1
  cfblk6/1 -> cfblk2/1
  cfblk8/1 -> cfblk3/1
  cfblk1/1 -> cfblk5/2
  cfblk3/1 -> cfblk6/1
  cfblk5/1 -> cfblk4/2
  cfblk4/1 -> cfblk9/1
  cfblk9/1 -> cfblk5/1

== system model/cfblk29/cfblk12 ==
  cfblk1 : Inport
  cfblk10 : Delay  SampleTime=1
  cfblk3 : simulink/Discrete/Transfer Fcn First Order  PoleZ=0.95  ICPrevOutput=0.0  DoSatur=off
  cfblk4 : simulink/Discrete/Difference  ICPrevInput=0.0  OutMin=[]  OutMax=[]  OutDataTypeStr=Inherit: Inherit via back propagation  OutDataType=fixdt(1, 16)  OutScaling=2^-10  DoSatur=off
  cfblk5 : Sin  TimeSource=Use external signal  SampleTime=0
  cfblk6 : Squeeze
  cfblk7 : Sqrt  Operator=rSqrt  AlgorithmType=Newton-Raphson
  cfblk8 : simulink/Math Operations/Slider Gain  gain=1  low=0  high=2
  cfblk9 : Sum  Inputs=|++
  cfblk2 : Outport
  wires:
  cfblk9/1 -> cfblk6/1
  cfblk1/1 -> cfblk8/1, cfblk7/1
  cfblk8/1 -> cfblk3/1
  cfblk5/1 -> cfblk9/1
  cfblk7/1 -> cfblk5/1
  cfblk6/1 -> cfblk4/1
  cfblk3/1 -> cfblk2/1
  cfblk4/1 -> cfblk10/1
  cfblk10/1 -> cfblk9/2

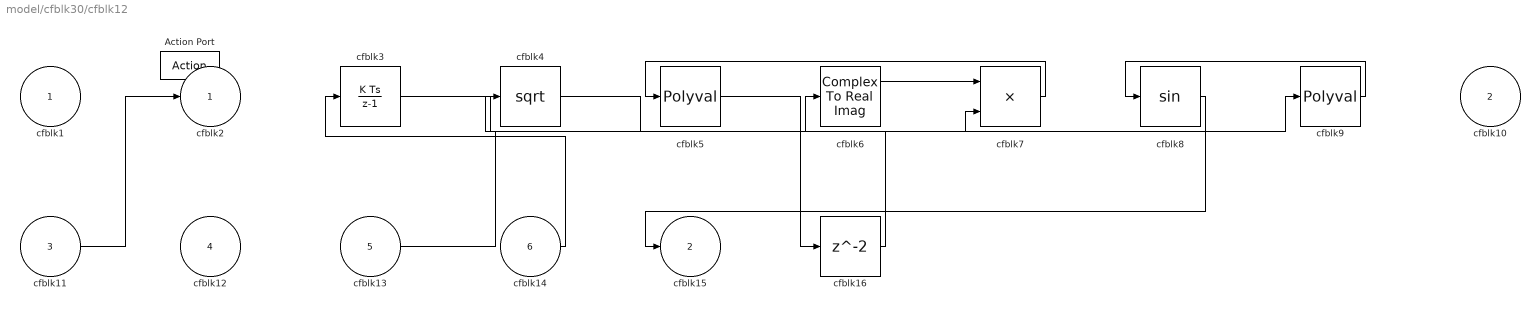
== system model/cfblk30/cfblk12 ==
  cfblk1 : Inport
  cfblk10 : Inport  Port=2
  cfblk11 : Inport  Port=3
  cfblk12 : Inport  Port=4
  cfblk13 : Inport  Port=5
  cfblk14 : Inport  Port=6
  Action Port : ActionPort  ActionPortLabel=if(u1 >= 0)
  cfblk16 : Delay
  cfblk3 : DiscreteIntegrator  SampleTime=-1  ICPrevOutput=DiscIntNeverNeededParam  ICPrevScaledInput=DiscIntNeverNeededParam
  cfblk4 : Sqrt
  cfblk5 : Polyval  Coefs=[ +2.081618890e-019, -1.441693666e-014, +4.719686976e-010, -8.536869453e-006, +1.621573104e-001, -8.087801117e+001 ]
  cfblk6 : ComplexToRealImag
  cfblk7 : Product  Inputs=**
  cfblk8 : Trigonometry
  cfblk9 : Polyval  Coefs=[ +2.081618890e-019, -1.441693666e-014, +4.719686976e-010, -8.536869453e-006, +1.621573104e-001, -8.087801117e+001 ]
  cfblk2 : Outport
  cfblk15 : Outport  Port=2
  wires:
  cfblk9/1 -> cfblk8/1
  cfblk3/1 -> cfblk9/1
  cfblk8/1 -> cfblk15/1
  cfblk7/1 -> cfblk5/1
  cfblk14/1 -> cfblk3/1
  cfblk13/1 -> cfblk6/1
  cfblk6/1 -> cfblk7/1
  cfblk11/1 -> cfblk2/1
  cfblk4/1 -> cfblk7/2
  cfblk5/1 -> cfblk16/1
  cfblk16/1 -> cfblk4/1
